simulink model "bank_housing"  (R2020a)
settings: Solver=VariableStepAuto  StartTime=0.0  StopTime=10.0  RelTol=1e-3
values from neighbouring files (symbols this model uses):
  D_0 = 1    [housing.m]
  i = 0.04    [housing.m]
  T_b = 1    [housing.m]
  T_d = 20    [housing.m]
  T_f = 0.5    [a_1.m]    (also in a_2.m; a_loss_function.m; bank_and_economy.m; bank_centralbank.m)
  T_h = 0.1    [a_1.m]    (also in a_2.m; a_loss_function.m; bank_and_economy.m; bank_centralbank.m)
settings Model: Creator=erlended  LastModifiedBy=erlended

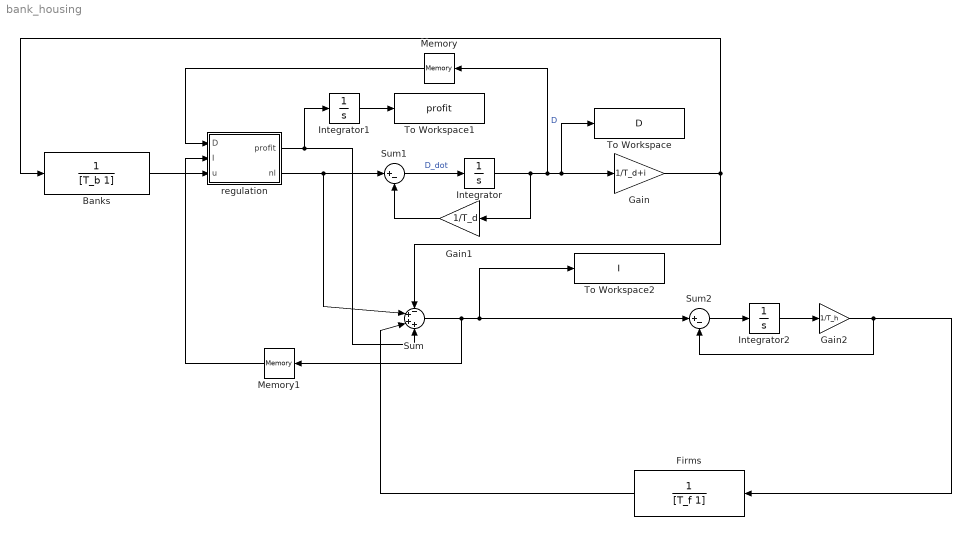
== system bank_housing ==
  Banks : TransferFcn  Denominator=[T_b 1]
  Firms : TransferFcn  Denominator=[T_f 1]
  Gain : Gain  Gain=1/T_d+i
  Gain1 : Gain  Gain=1/T_d
  Gain2 : Gain  Gain=1/T_h
  Integrator : Integrator  InitialCondition=D_0
  Integrator1 : Integrator
  Integrator2 : Integrator  InitialCondition=D_0
  Memory : Memory
  Memory1 : Memory
  Sum : Sum  Inputs=-+++
  Sum1 : Sum  Inputs=|+-
  Sum2 : Sum  Inputs=|+-
  To Workspace : ToWorkspace  VariableName=D  SaveFormat=Timeseries  SampleTime=-1
  To Workspace1 : ToWorkspace  VariableName=profit  SaveFormat=Timeseries  SampleTime=-1
  To Workspace2 : ToWorkspace  VariableName=I  SaveFormat=Timeseries  SampleTime=-1
  regulation : MATLAB Function  TreatAsAtomicUnit=on
  wires:
  Integrator/1 -> Gain1/1, Memory/1, To Workspace/1, Gain/1  "D"
  Gain/1 -> Sum/1, Banks/1
  Gain2/1 -> Sum2/2, Firms/1
  Sum/1 -> Memory1/1, Sum2/1, To Workspace2/1
  Firms/1 -> Sum/3
  Sum1/1 -> Integrator/1  "D_dot"
  Gain1/1 -> Sum1/2
  Banks/1 -> regulation/3(u)
  regulation/2(nl) -> Sum/2, Sum1/1
  regulation/1(profit) -> Sum/4, Integrator1/1
  Integrator1/1 -> To Workspace1/1
  Memory/1 -> regulation/1(D)
  Memory1/1 -> regulation/2(I)
  Integrator2/1 -> Gain2/1
  Sum2/1 -> Integrator2/1

== matlab function bank_housing/regulation ==
  data: profit output; D input; I input; u input; nl output
function [profit, nl]= fcn(D, I, u)
diff = 5*I-D;
nl = u;
profit = 0;
if D > 5*I
    nl = 0;
    profit = u;
elseif u <= diff
    nl = u; 
    profit = 0;
else
    nl = diff;
    profit = u - diff; 
end
